simulink model "pendubot_simulate_1_8_5_2017_fuzzy"  (Simulink 8.0)
settings: Solver=ode3  StartTime=0.0  StopTime=100  FixedStep=0.01  RelTol=1e-3
values from neighbouring files (symbols this model uses):
  a1 = par(pop_index,1)    [pidGA.m]
  a2 = par(pop_index,2)    [pidGA.m]
  c1 = par(pop_index,3)    [pidGA.m]
  c2 = par(pop_index,4)    [pidGA.m]
  k2 = par(pop_index,5)    [pidGA.m]
  nuy2 = par(pop_index,6)    [pidGA.m]
  q1_dot_init = 0.1    [pidGA.m]
  q1_init = pi/2+0.1    (= 1.67079632679)    [pidGA.m]
  q2_dot_init = -0.2    [pidGA.m]
  q2_init = -0.1    [pidGA.m]
settings Model: Creator=donghai  LastModifiedBy=donghai

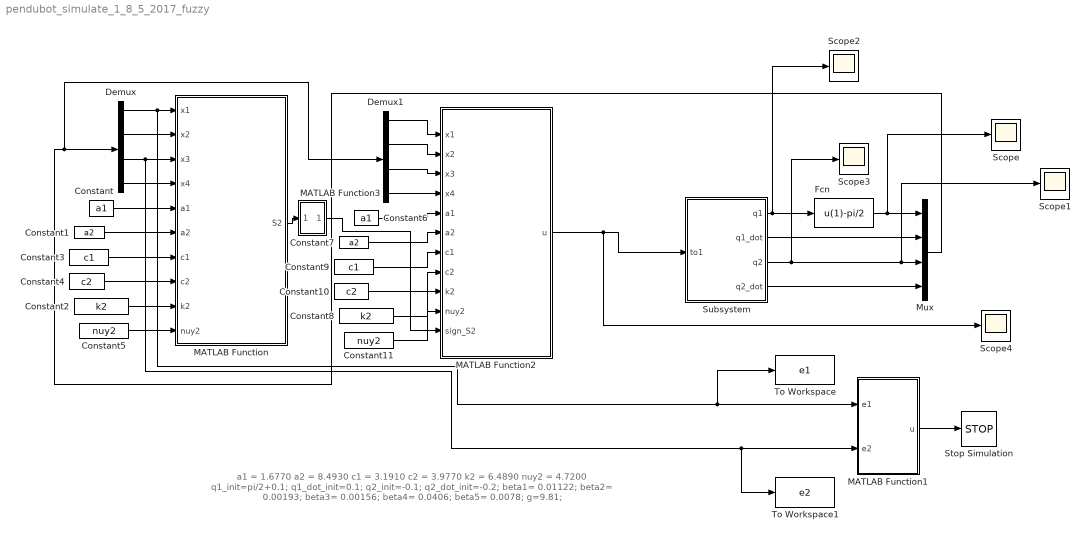
== system pendubot_simulate_1_8_5_2017_fuzzy ==
  note: a1 =    1.6770
      | a2 =    8.4930
      | c1 =    3.1910
      | c2 =    3.9770
      | k2 =    6.4890
      | nuy2 =    4.7200
      |
      | q1_init=pi/2+0.1;
      | q1_dot_init=0.1;
      | q2_init=-0.1;
      | q2_dot_init=-0.2;
      |
      | beta1= 0.01122;
      | beta2= 0.00193;
      | beta3= 0.00156;
      | beta4= 0.0406;
      | beta5= 0.0078;
      | g=9.81;
  Constant : Constant  Value=a1
  Constant1 : Constant  Value=a2
  Constant10 : Constant  Value=c2
  Constant11 : Constant  Value=nuy2
  Constant2 : Constant  Value=k2
  Constant3 : Constant  Value=c1
  Constant4 : Constant  Value=c2
  Constant5 : Constant  Value=nuy2
  Constant6 : Constant  Value=a1
  Constant7 : Constant  Value=a2
  Constant8 : Constant  Value=k2
  Constant9 : Constant  Value=c1
  Demux : Demux
  Demux1 : Demux
  Fcn : Fcn  Expr=u(1)-pi/2
  MATLAB Function : MATLAB Function  TreatAsAtomicUnit=on
  MATLAB Function1 : MATLAB Function  TreatAsAtomicUnit=on
  MATLAB Function2 : MATLAB Function  TreatAsAtomicUnit=on
  MATLAB Function3 : MATLAB Function  TreatAsAtomicUnit=on
  Mux : Mux
  Scope{,1..4} (5 alike) : Scope
      Scope2 settings: SaveName=ScopeData2
      Scope3 settings: SaveName=ScopeData3
      Scope4 settings: SaveName=ScopeData4
  Stop Simulation : Stop
  Subsystem : Subsystem
  To Workspace : ToWorkspace  VariableName=e1  SampleTime=-1
  To Workspace1 : ToWorkspace  VariableName=e2  SampleTime=-1
  wires:
  Subsystem/1(q1) -> Scope2/1, Fcn/1
  Demux/1 -> To Workspace/1, MATLAB Function1/1(e1), MATLAB Function/1(x1)
  Demux/2 -> MATLAB Function/2(x2)
  Demux/3 -> To Workspace1/1, MATLAB Function1/2(e2), MATLAB Function/3(x3)
  Demux/4 -> MATLAB Function/4(x4)
  Fcn/1 -> Scope/1, Mux/1
  Subsystem/2(q1_dot) -> Mux/2
  Subsystem/3(q2) -> Scope3/1, Scope1/1, Mux/3
  Subsystem/4(q2_dot) -> Mux/4
  Mux/1 -> Demux1/1, Demux/1
  Constant/1 -> MATLAB Function/5(a1)
  Constant1/1 -> MATLAB Function/6(a2)
  Constant3/1 -> MATLAB Function/7(c1)
  Constant4/1 -> MATLAB Function/8(c2)
  Constant2/1 -> MATLAB Function/9(k2)
  Constant5/1 -> MATLAB Function/10(nuy2)
  MATLAB Function1/1(u) -> Stop Simulation/1
  Demux1/1 -> MATLAB Function2/1(x1)
  Demux1/2 -> MATLAB Function2/2(x2)
  Demux1/3 -> MATLAB Function2/3(x3)
  Demux1/4 -> MATLAB Function2/4(x4)
  Constant6/1 -> MATLAB Function2/5(a1)
  Constant7/1 -> MATLAB Function2/6(a2)
  Constant9/1 -> MATLAB Function2/7(c1)
  Constant10/1 -> MATLAB Function2/8(c2)
  Constant8/1 -> MATLAB Function2/9(k2)
  Constant11/1 -> MATLAB Function2/10(nuy2)
  MATLAB Function/1(S2) -> MATLAB Function3/1(in)
  MATLAB Function3/1(out) -> MATLAB Function2/11(sign_S2)
  MATLAB Function2/1(u) -> Scope4/1, Subsystem/1(to1)

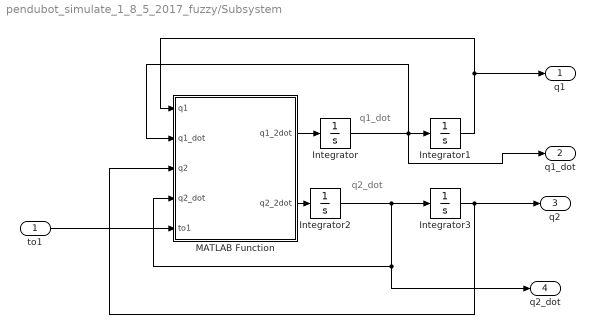
== system pendubot_simulate_1_8_5_2017_fuzzy/Subsystem ==
  note: q2_dot
  note: q1_dot
  to1 : Inport
  Integrator : Integrator  InitialCondition=q1_dot_init
  Integrator1 : Integrator  InitialCondition=q1_init
  Integrator2 : Integrator  InitialCondition=q2_dot_init
  Integrator3 : Integrator  InitialCondition=q2_init
  MATLAB Function : MATLAB Function  TreatAsAtomicUnit=on
  q1 : Outport
  q1_dot : Outport  Port=2
  q2 : Outport  Port=3
  q2_dot : Outport  Port=4
  wires:
  MATLAB Function/1(q1_2dot) -> Integrator/1
  Integrator/1 -> MATLAB Function/2(q1_dot), q1_dot/1, Integrator1/1
  Integrator1/1 -> q1/1, MATLAB Function/1(q1)
  MATLAB Function/2(q2_2dot) -> Integrator2/1
  Integrator2/1 -> q2_dot/1, MATLAB Function/4(q2_dot), Integrator3/1
  Integrator3/1 -> q2/1, MATLAB Function/3(q2)
  to1/1 -> MATLAB Function/5(to1)

== matlab function MATLAB Function ==
  data: S2 output double; x1 input double; x2 input double; x3 input double; x4 input double; a1 input double; a2 input double; c1 input double; c2 input double; k2 input double; nuy2 input double
function S2 = fcn(x1,x2,x3,x4,a1,a2,c1,c2,k2,nuy2)
beta1= 0.01122;
beta2= 0.00193;
beta3= 0.00156;
beta4= 0.0406;
beta5= 0.0078;
g=9.81;

f1=1/(beta1*beta2-beta3^3*(cos(x3))^2)*(beta2*0+beta2*beta3*(x2+x4)^2*sin(x3)+beta3^2*x2^2*sin(x3)*cos(x3)-beta2*beta4*g*cos((x1+pi/2))+beta3*beta5*g*cos(x3)*cos((x1+pi/2)+x3));
f2=1/(beta1*beta2-beta3^3*(cos(x3))^2)*((-beta2-beta3*cos(x3))*0-beta3*(beta2+beta3*cos(x3))*(x2+x4)^2*sin(x3)-beta5*g*(beta1+beta3*cos(x3))*cos((x1+pi/2)+x3)+beta4*g*(beta2+beta3*cos(x3))*cos((x1+pi/2))-beta3*x2^2*sin(x3)*(beta1+beta3*cos(x3)));

% b1=(x2_dot-f1)/to1; b1=simple(b1)
% b2=(x4_dot-f2)/to1; b2=simple(b2)

b1 = beta2/(beta1*beta2 - beta3^3*cos(x3)^2);
b2 =-(beta2 + beta3*cos(x3))/(beta1*beta2 - beta3^3*cos(x3)^2);

s1=c1*x1+x2;   %i=1
s2=c2*x3+x4;   %i=2

u_eq_1=-(c1*x2+f1)/b1;
u_eq_2=-(c2*x4+f2)/b2;

S1=a1*s1;
S2=(a1*a2)*s1+(a2)*s2;

% u=(((a1*a2)*b1*u_eq_1+(a2)*b2*u_eq_2)-(k2*S2+nuy2*sign(S2)))/((a1*a2)*b1+(a2)*b2);

== matlab function Subsystem/MATLAB Function ==
  data: q1 input double; q1_2dot output double; q1_dot input double; q2 input double; q2_dot input double; to1 input double; q2_2dot output double
function [q1_2dot,q2_2dot] = fcn(q1, q1_dot,q2,q2_dot,to1)
beta1=0.01122;
beta2=0.00193;
beta3=0.00156;
beta4=0.0406;
beta5=0.0078;
g=9.81;
q1_2dot=1/(beta1*beta2-beta3^3*(cos(q2))^2)*(beta2*to1+beta2*beta3*(q1_dot+q2_dot)^2*sin(q2)+beta3^2*q1_dot^2*sin(q2)*cos(q2)-beta2*beta4*g*cos(q1)+beta3*beta5*g*cos(q2)*cos(q1+q2));
q2_2dot=1/(beta1*beta2-beta3^3*(cos(q2))^2)*((-beta2-beta3*cos(q2))*to1-beta3*(beta2+beta3*cos(q2))*(q1_dot+q2_dot)^2*sin(q2)-beta5*g*(beta1+beta3*cos(q2))*cos(q1+q2)+beta4*g*(beta2+beta3*cos(q2))*cos(q1)-beta3*q1_dot^2*sin(q2)*(beta1+beta3*cos(q2)));

== matlab function MATLAB Function1 ==
  data: u output double; e1 input double; e2 input double
function u = fcn(e1,e2)
if ((abs(e1)>5)||(abs(e2)>5))
    u=1;
else
    u=0;
end

== matlab function MATLAB Function2 ==
  data: u output double; x1 input double; x2 input double; x3 input double; x4 input double; a1 input double; a2 input double; c1 input double; c2 input double; k2 input double; nuy2 input double; sign_S2 input double
function u = fcn(x1,x2,x3,x4,a1,a2,c1,c2,k2,nuy2,sign_S2)
beta1= 0.01122;
beta2= 0.00193;
beta3= 0.00156;
beta4= 0.0406;
beta5= 0.0078;
g=9.81;

f1=1/(beta1*beta2-beta3^3*(cos(x3))^2)*(beta2*0+beta2*beta3*(x2+x4)^2*sin(x3)+beta3^2*x2^2*sin(x3)*cos(x3)-beta2*beta4*g*cos((x1+pi/2))+beta3*beta5*g*cos(x3)*cos((x1+pi/2)+x3));
f2=1/(beta1*beta2-beta3^3*(cos(x3))^2)*((-beta2-beta3*cos(x3))*0-beta3*(beta2+beta3*cos(x3))*(x2+x4)^2*sin(x3)-beta5*g*(beta1+beta3*cos(x3))*cos((x1+pi/2)+x3)+beta4*g*(beta2+beta3*cos(x3))*cos((x1+pi/2))-beta3*x2^2*sin(x3)*(beta1+beta3*cos(x3)));

% b1=(x2_dot-f1)/to1; b1=simple(b1)
% b2=(x4_dot-f2)/to1; b2=simple(b2)

b1 = beta2/(beta1*beta2 - beta3^3*cos(x3)^2);
b2 =-(beta2 + beta3*cos(x3))/(beta1*beta2 - beta3^3*cos(x3)^2);

s1=c1*x1+x2;   %i=1
s2=c2*x3+x4;   %i=2

u_eq_1=-(c1*x2+f1)/b1;
u_eq_2=-(c2*x4+f2)/b2;

S1=a1*s1;
S2=(a1*a2)*s1+(a2)*s2;

u=(((a1*a2)*b1*u_eq_1+(a2)*b2*u_eq_2)-(k2*S2+nuy2*sign_S2))/((a1*a2)*b1+(a2)*b2);

== matlab function MATLAB Function3 ==
  data: out output double; in input double
function out = fcn(in)
if in>1
    out=1;
elseif in<-1
    out=-1;
else
    out=in;
end
